simulink model "single_phase_bridge_lr"  (Simulink 6.1)
settings: Solver=ode23tb  StartTime=0.0  StopTime=0.2999  MaxStep=1e-4  RelTol=1e-3  AbsTol=.01
libraries: powerlib x9
settings Model: LastModifiedBy=ThinkPad
settings DebuggingCC: SolverPrmCheckMsg=warning

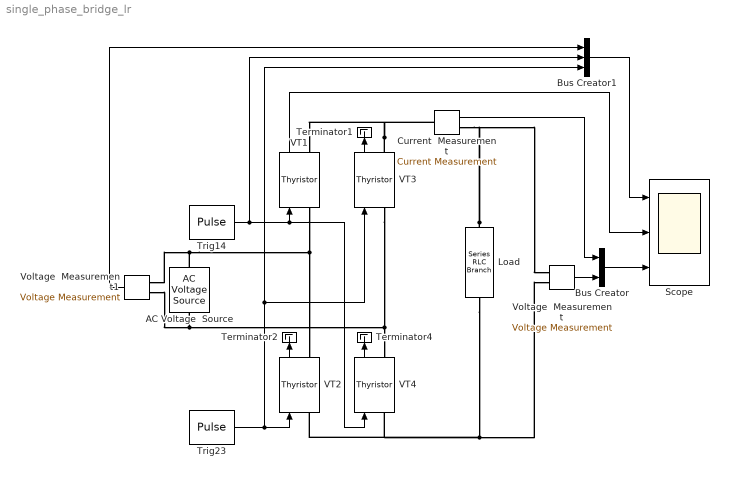
== system single_phase_bridge_lr ==
  AC Voltage  Source : powerlib/Electrical Sources/AC Voltage Source  Orientation=up  Amplitude=100  Phase=0  Frequency=50  SampleTime=0  Measurements=None
  Bus Creator : BusCreator  DialogController=Simulink.DDGSource_Bus  Inputs=2
  Bus Creator1 : BusCreator  DialogController=Simulink.DDGSource_Bus  Inputs=3
  Current  Measurement : powerlib/Measurements/Current Measurement  PhasorSimulation=off  OutputType=Complex  PSBequivalent=0
  Load : powerlib/Elements/Series RLC Branch  Orientation=down  PhysicalDomain=powersysdomain  SubClassName=unknown  LeftPortType=p1  RightPortType=p1  LConnTagsString=__new0  RConnTagsString=__new0  Resistance=1  Inductance=0.1  Capacitance=inf  Measurements=None
  Scope : Scope  NumInputPorts=3
      settings: TimeRange=0.1  YMin=-100~-100~-100  YMax=100~100~100  Decimation=5  SampleInput=on  SampleTime=1e-4
  Terminator1 : Terminator
      settings: Orientation=up
  Terminator2 : Terminator
      settings: Orientation=up
  Terminator4 : Terminator
      settings: Orientation=up
  Trig14 : DiscretePulseGenerator  PulseType=Time based  Amplitude=10  Period=0.02  PulseWidth=5  PhaseDelay=0.0025
  Trig23 : DiscretePulseGenerator  PulseType=Time based  Amplitude=10  Period=0.02  PulseWidth=5  PhaseDelay=0.0125
  VT{1..4} (4 alike) : powerlib/Power Electronics/Thyristor  Orientation=up  Ron=0.01  Lon=0  Vf=0.8  IC=0  Rs=1000  Cs=100e-9  Measurements=on
  Voltage  Measurement : powerlib/Measurements/Voltage Measurement  PhasorSimulation=off  OutputType=Complex  PSBequivalent=0
  Voltage  Measurement1 : powerlib/Measurements/Voltage Measurement  Orientation=left  PhasorSimulation=off  OutputType=Complex  PSBequivalent=0
  wires:
  Trig14/1 -> VT1/1, VT4/1, Bus Creator1/2
  VT1/1 -> Scope/2
  Voltage  Measurement/1 -> Bus Creator/2
  Bus Creator/1 -> Scope/3
  Current  Measurement/1 -> Bus Creator/1
  Trig23/1 -> VT2/1, VT3/1, Bus Creator1/3
  Bus Creator1/1 -> Scope/1
  Voltage  Measurement1/1 -> Bus Creator1/1
  VT3/1 -> Terminator1/1
  VT2/1 -> Terminator2/1
  VT4/1 -> Terminator4/1
  connections:
  Current  Measurement/RConn1 -- Load/LConn1 -- Voltage  Measurement/LConn1
  Current  Measurement/LConn1 -- VT1/RConn1 -- VT3/RConn1
  VT2/LConn1 -- VT4/LConn1 -- Voltage  Measurement/LConn2 -- Load/RConn1
  Voltage  Measurement1/LConn2 -- VT3/LConn1 -- VT4/RConn1 -- AC Voltage  Source/LConn1
  Voltage  Measurement1/LConn1 -- VT1/LConn1 -- VT2/RConn1 -- AC Voltage  Source/RConn1
